simulink model "Two_Level_SVM_No_PV_No_Control_Sw_Benchmark_v2"  (R2022b)
settings: Solver=FixedStepAuto  StartTime=0.0  StopTime=5  FixedStep=1e-7  RelTol=1e-3
model workspace (MAT data in the model file):
  Phase_Shift : Simulink.Parameter (value not decoded)
  Vrms_p : Simulink.Parameter (value not decoded)
symbols that are objects in the model workspace (value not decoded): Phase_Shift, Vrms_p
libraries: spsIGBTDiodeLib x6, slpidlib x5, spsThreePhaseVIMeasurementLib x5, spsThreePhaseSeriesRLCBranchLib x4, spsGroundLib x2, spsabctodq0Lib x2, spsdq0toabcLib x1, spsDCVoltageSourceLib x1, spsThreePhaseProgrammableVoltageSourceLib x1, eeGeneralControl x1, spsabctoAlphaBetaZeroLib x1, eePwmGeneratorTwoLevel x1
(part 2 of 2)

== matlab function Two_Level_SVM_No_PV_No_Control_Sw_Benchmark_v2/SVM3phaseC ==
  data: Vr_ll input; duration output; Vdc input; Ts input; outputStates output; sz1 output; s1 output; s2 output; sz2 output
% Switching Function Generation
% Inputs: 
%   - terminal voltage reference in abc
%   - DC Link Voltage
% Intermediate Outputs:
%   - 1st z switch state set
%   - 1st nz switch state set
%   - 2nd nz switch state set
%   - 2nd z switch state set
% Outputs:
%   - duration column vector with seven durations [T0/4; T1/2; T2/2; T0/2;
%     T2/2; T1/2; T0/4]
%   - output switching states 7x3 matrix; each row has switching state for
%     three phase legs for corresponding time
%  
 
%   - z state duty cycle
%   - 1st nz state duty cycle
%   - 2nd nz state duty cycle
 
 
function [duration, outputStates, sz1, s1, s2, sz2] = getSVM3phaseC( Vr_ll, Vdc, Ts )
    
    % Guarantee outputs are assigned
    sz1 = zeros(3,1); s1 = zeros(3,1); s2 = zeros(3,1); s3 = zeros(3,1);
    dz = 0; d1 = 0; d2 = 0; d3 = 0;
    % Define the reference frame transformation
    Taby = sqrt(2/3)*[1 -.5 -.5; 0 sqrt(3)/2 -sqrt(3)/2; 1/2 1/2 1/2];
    
    % SVM Implementation Definitions: /////////////////////////////////////
    % ///////////////////////////////////////////////////////////////////
    % ///////////////////////////////////////////////////////////////////
    % ///////////////////////////////////////////////////////////////////
    % ///////////////////////////////////////////////////////////////////
    
    
    % Define the switch state vectors
    % Columns are separate vectors (i.e. 8 vectors), rows are separate
    % phase legs (i.e. 3 legs)
    % Note that the same order is used for all following definitions and
    % column indices are used to cross reference switch state vectors
    % order is [Sa, Sb, Sc]
    states = [...
        [ 1 1 1 ]', [ 1 0 0 ]', [ 1 1 0 ]', [ 0 1 0 ]',...% ppp pnn ppn npn
        [ 0 1 1 ]', [ 0 0 1 ]', [ 1 0 1 ]', [ 0 0 0 ]'];  % npp nnp pnp nnn
    
 
    % Define the Switching Vectors in AB,BC,CA coord.
    Vsv_ll = [...
        Vdc*[ 0  0  0]', Vdc*[ 1 0 -1]', Vdc*[ 0 1 -1]', Vdc*[ -1  1 0 ]'...% ppp pnn ppn npn
        Vdc*[-1  0 1]', Vdc*[0 -1 1]', Vdc*[1 -1  0]', Vdc*[ 0 0 0]']; % npp nnp pnp nnn
    
    % Convert to aby coord. switch state vectors
    Vsv_aby = zeros(3,8);
    for i=1:8
        Vsv_aby(:,i) = Taby*Vsv_ll(:,i);
    end
    
    % Define vector pairs: a non-zero vector paired with the nearest zero
    % vector
    %   1st col = nz vector column index, 2nd col = corresponding z vector
    %   column index
    %   allows look up in the states and Vsv_aby arrays
    nzAndZVectorPairs = [ 2, 8; 3, 1; 4, 8; 5, 1; 6, 8; 7, 1];
 
    % Define the Sectors
    % rows are sectors
    Sectors = [...
        [2 3]'; %sector 1, pnn, ppn
        [3 4]'; %sector 2, ppn, npn
        [4 5]'; %sector 3, npn, npp
        [5 6]'; %sector 4, npp, nnp
        [6 7]'; %sector 5, nnp, pnp
        [7 2]']; %sector 6, pnp, pnn
  
    
    
    % Convert reference vector to aby
    Vr_aby = Taby*Vr_ll;
    
    
    % Sector Identification /////////////////////////////////////////////
    % ///////////////////////////////////////////////////////////////////
    % ///////////////////////////////////////////////////////////////////
    % ///////////////////////////////////////////////////////////////////
    
    
    % Calculate Vr angle on alpha beta plane
    % If the alpha, beta vectors of Vr are zero, arbitrarily set angle to 0
    if Vr_aby(1) == 0 && Vr_aby(2) == 0
        th1_aby = 0;
    else
        if Vr_aby(1) >= 0 && Vr_aby(2) >= 0
            th1_aby = atan(Vr_aby(2)/Vr_aby(1))*180/pi;
        elseif Vr_aby(1) < 0 && Vr_aby(2) >= 0
            th1_aby = atan(Vr_aby(2)/Vr_aby(1))*180/pi + 180;
        elseif Vr_aby(1) < 0 && Vr_aby(2) < 0
            th1_aby = atan(Vr_aby(2)/Vr_aby(1))*180/pi + 180;
        else
            th1_aby = atan(Vr_aby(2)/Vr_aby(1))*180/pi + 360;
        end
    end
    % Select sector based on angle
    if th1_aby >= 30.0 && th1_aby < 90.0
        currS = 1;
    elseif th1_aby >= 90.0 && th1_aby < 150.0
        currS = 2;
    elseif th1_aby >= 150.0 && th1_aby < 210.0
        currS = 3;
    elseif th1_aby >= 210.0 && th1_aby < 270.0
        currS = 4;
    elseif th1_aby >= 270.0 && th1_aby < 330.0
        currS = 5;
    else
        currS = 6;
    end
 
   % Now currS has sector
    
    % Calculation of switch state vector duty cycles //////////////////////
    % ///////////////////////////////////////////////////////////////////
    % ///////////////////////////////////////////////////////////////////
    % ///////////////////////////////////////////////////////////////////
 
    % get the current sector switching state vectors in aby coordinates
    current_sector_vectors = Sectors(2*currS-1:2*currS,1);
    % Start with (0, 0, 0) every time, i.e., state 8

    if currS == 1 || currS == 3 || currS == 5
        V1_aby = Vsv_aby(:,current_sector_vectors(1)); s1 = states(:,current_sector_vectors(1));
        V2_aby = Vsv_aby(:,current_sector_vectors(2)); s2 = states(:,current_sector_vectors(2));
    else
        V1_aby = Vsv_aby(:,current_sector_vectors(2)); s1 = states(:,current_sector_vectors(2));
        V2_aby = Vsv_aby(:,current_sector_vectors(1)); s2 = states(:,current_sector_vectors(1));
    end
    
    % Don't need anymore since the first 0 vector is state 8
%     % identify 1st Z vector
%     % lookup in nzAndZVectorPairs array
%     for i=1:length(nzAndZVectorPairs)
%         if nzAndZVectorPairs(i,1) == current_sector_vectors(1)
%             sz1 = states(:,nzAndZVectorPairs(i,2));
%         end
%     end
    
    % get the switching vector duty cycles 
    d_12 = inv(V1_aby(1:2)*[1 0] + V2_aby(1:2)*[0 1])*Vr_aby(1:2);
    dz = 1 - d_12(1) - d_12(2);
    d1 = d_12(1); 
    d2 = d_12(2);

    % get the duration and output switching states for 3 phase centered
    duration = [dz/4;d1/2;d2/2;dz/2;d2/2;d1/2;dz/4]*Ts;

    % get zero vector states
%     if sz1 == [0;0;0]
%         sz2 = [1;1;1];
%     else
%         sz2 = [0;0;0];
%     end
    sz1 = [0;0;0];
    sz2 = [1;1;1];
    
    % get output switching states
    outputStates = [sz1 s1 s2 sz2 s2 s1 sz1];

== matlab function Two_Level_SVM_No_PV_No_Control_Sw_Benchmark_v2/MATLAB Function ==
  data: Vr_ll input; duration output; Vdc input; Ts input; outputStates output; sz1 output; s1 output; s2 output; sz2 output
function [duration, outputStates, sz1, s1, s2, sz2] = getSVM3phaseC( Vr_ll, Vdc, Ts )
    
    % Guarantee outputs are assigned
    sz1 = zeros(3,1); s1 = zeros(3,1); s2 = zeros(3,1); s3 = zeros(3,1);
    dz = 0; d1 = 0; d2 = 0; d3 = 0;
    % Define the reference frame transformation
    Taby = sqrt(2/3)*[1 -.5 -.5; 0 sqrt(3)/2 -sqrt(3)/2; 1/2 1/2 1/2];
    
    % SVM Implementation Definitions: /////////////////////////////////////
    % ///////////////////////////////////////////////////////////////////
    % ///////////////////////////////////////////////////////////////////
    % ///////////////////////////////////////////////////////////////////
    % ///////////////////////////////////////////////////////////////////
    
    
    % Define the switch state vectors
    % Columns are separate vectors (i.e. 8 vectors), rows are separate
    % phase legs (i.e. 3 legs)
    % Note that the same order is used for all following definitions and
    % column indices are used to cross reference switch state vectors
    % order is [Sa, Sb, Sc]
    states = [...
        [ 1 1 1 ]', [ 1 0 0 ]', [ 1 1 0 ]', [ 0 1 0 ]',...% ppp pnn ppn npn
        [ 0 1 1 ]', [ 0 0 1 ]', [ 1 0 1 ]', [ 0 0 0 ]'];  % npp nnp pnp nnn
    
 
    % Define the Switching Vectors in AB,BC,CA coord.
    Vsv_ll = [...
        Vdc*[ 0  0  0]', Vdc*[ 1 0 -1]', Vdc*[ 0 1 -1]', Vdc*[ -1  1 0 ]'...% ppp pnn ppn npn
        Vdc*[-1  0 1]', Vdc*[0 -1 1]', Vdc*[1 -1  0]', Vdc*[ 0 0 0]']; % npp nnp pnp nnn
    
    % Convert to aby coord. switch state vectors
    Vsv_aby = zeros(3,8);
    for i=1:8
        Vsv_aby(:,i) = Taby*Vsv_ll(:,i);
    end
    
    % Define vector pairs: a non-zero vector paired with the nearest zero
    % vector
    %   1st col = nz vector column index, 2nd col = corresponding z vector
    %   column index
    %   allows look up in the states and Vsv_aby arrays
    nzAndZVectorPairs = [ 2, 8; 3, 1; 4, 8; 5, 1; 6, 8; 7, 1];
 
    % Define the Sectors
    % rows are sectors
    Sectors = [...
        [2 3]'; %sector 1, pnn, ppn
        [3 4]'; %sector 2, ppn, npn
        [4 5]'; %sector 3, npn, npp
        [5 6]'; %sector 4, npp, nnp
        [6 7]'; %sector 5, nnp, pnp
        [7 2]']; %sector 6, pnp, pnn
  
    
    
    % Convert reference vector to aby
    Vr_aby = Taby*Vr_ll;
    
    
    % Sector Identification /////////////////////////////////////////////
    % ///////////////////////////////////////////////////////////////////
    % ///////////////////////////////////////////////////////////////////
    % ///////////////////////////////////////////////////////////////////
    
    
    % Calculate Vr angle on alpha beta plane
    % If the alpha, beta vectors of Vr are zero, arbitrarily set angle to 0
    if Vr_aby(1) == 0 && Vr_aby(2) == 0
        th1_aby = 0;
    else
        if Vr_aby(1) >= 0 && Vr_aby(2) >= 0
            th1_aby = atan(Vr_aby(2)/Vr_aby(1))*180/pi;
        elseif Vr_aby(1) < 0 && Vr_aby(2) >= 0
            th1_aby = atan(Vr_aby(2)/Vr_aby(1))*180/pi + 180;
        elseif Vr_aby(1) < 0 && Vr_aby(2) < 0
            th1_aby = atan(Vr_aby(2)/Vr_aby(1))*180/pi + 180;
        else
            th1_aby = atan(Vr_aby(2)/Vr_aby(1))*180/pi + 360;
        end
    end
    % Select sector based on angle
    if th1_aby >= 30.0 && th1_aby < 90.0
        currS = 1;
    elseif th1_aby >= 90.0 && th1_aby < 150.0
        currS = 2;
    elseif th1_aby >= 150.0 && th1_aby < 210.0
        currS = 3;
    elseif th1_aby >= 210.0 && th1_aby < 270.0
        currS = 4;
    elseif th1_aby >= 270.0 && th1_aby < 330.0
        currS = 5;
    else
        currS = 6;
    end
 
   % Now currS has sector
    
    % Calculation of switch state vector duty cycles //////////////////////
    % ///////////////////////////////////////////////////////////////////
    % ///////////////////////////////////////////////////////////////////
    % ///////////////////////////////////////////////////////////////////
 
    % get the current sector switching state vectors in aby coordinates
    current_sector_vectors = Sectors(2*currS-1:2*currS,1);
    V1_aby = Vsv_aby(:,current_sector_vectors(1)); s1 = states(:,current_sector_vectors(1));
    V2_aby = Vsv_aby(:,current_sector_vectors(2)); s2 = states(:,current_sector_vectors(2));
    
    % identify 1st Z vector
    % lookup in nzAndZVectorPairs array
    for i=1:length(nzAndZVectorPairs)
        if nzAndZVectorPairs(i,1) == current_sector_vectors(1)
            sz1 = states(:,nzAndZVectorPairs(i,2));
        end
    end
 
    % get the switching vector duty cycles 
    d_12 = inv(V1_aby(1:2)*[1 0] + V2_aby(1:2)*[0 1])*Vr_aby(1:2);
    dz = 1 - d_12(1) - d_12(2);
    d1 = d_12(1); 
    d2 = d_12(2);

    % get the duration and output switching states for 3 phase centered
    duration = [dz/4;d1/2;d2/2;dz/2;d2/2;d1/2;dz/4]*Ts;

    % get second zero vector state
    if sz1 == [0;0;0]
        sz2 = [1;1;1];
    else
        sz2 = [0;0;0];
    end
    
    % get output switching states
    outputStates = [sz1'; s1'; s2'; sz2'; s2'; s1'; sz1'];

== matlab function Two_Level_SVM_No_PV_No_Control_Sw_Benchmark_v2/Measurements/MATLAB Function ==
  data: Uabc input; P output; Iabc input; Q output; U output
function [P,Q,U] = fcn(Uabc,Iabc)

Ua = Uabc(1);
Ub = Uabc(2);
Uc = Uabc(3);

Ia = Iabc(1);
Ib = Iabc(2);
Ic = Iabc(3);

P = Ua*Ia + Ub*Ib + Uc*Ic;
Q = 1/sqrt(3)*((Ua-Ub)*Ic + (Ub-Uc)*Ia + (Uc-Ua)*Ib);
U = sqrt(2)*sqrt(-Ua*Ub-Ub*Uc-Uc*Ua);

== matlab function Two_Level_SVM_No_PV_No_Control_Sw_Benchmark_v2/MATLAB Function1 ==
  data: t input; T_sw input; States output; duration input; states input
function States = fcn(t, T_sw, duration, states)

t = mod(t,T_sw);

t1 = duration(1,1);
t2 = duration(2,1);
t3 = duration(3,1);
t4 = duration(4,1);

% if t1 < 1e-6
%     t1 = 1e-6;
% elseif t2 < 1e-6
%     t2 = 1e-6;
% elseif t3 < 1e-6
%     t3 = 1e-6;
% elseif t4 < 1e-6
%     t4 = 1e-6;
% end


if t < t1
    States = states(1:3);
elseif t >= t1 && t < t1 + t2
    States = states(4:6);
elseif t >= t1 + t2 && t < t1 + t2 + t3
    States = states(7:9);
elseif t >= t1 + t2 + t3 && t < t1 + t2 + t3 + t4
    States = states(10:12);
elseif t >= t1 + t2 + t3 + t4 && t < t1 + t2 + 2*t3 + t4
    States = states(13:15);
elseif t >= t1 + t2 + 2*t3 + t4 && t < t1 + 2*t2 + 2*t3 + t4
    States = states(16:18);
else
    States = states(19:21);
end

== matlab function Two_Level_SVM_No_PV_No_Control_Sw_Benchmark_v2/MATLAB Function2 ==
  data: States input; g output
function g = fcn(States)

g = zeros(6,1);

g(1) = States(1);
g(3) = States(2);
g(5) = States(3);

if g(1) == 1
    g(2) = 0;
else
    g(2) = 1;
end

if g(3) == 1
    g(4) = 0;
else
    g(4) = 1;
end

if g(5) == 1
    g(6) = 0;
else
    g(6) = 1;
end
